simulink model "InterpolationIkinePD2019"  (R2019b)
settings: Solver=FixedStepDiscrete  StartTime=0.0  StopTime=inf  FixedStep=1/100  RelTol=1e-3
values from neighbouring files (symbols this model uses):
  Kd = 0.1    [LetterN.mat]    (also in initNew.m; panda.m)
  Kp = 10    [LetterN.mat]    (also in initNew.m; panda.m)
libraries: xpcutilitieslib x2, xpcrtudplib x2, robotcorelib x1, robotmaniplib x1, simulink x1
settings Model: EnablePacing=on  Creator=Aljaz  LastModifiedBy=jelac
settings DebuggingCC: ArithmeticOperatorsInVariantConditions=warning
settings SFSimCC: CustomCodeUndefinedFunction=UseInterfaceOnly
settings RTWCC: Toolchain=Microsoft Visual C++ 2019 v16.0 | nmake (64-bit Windows)

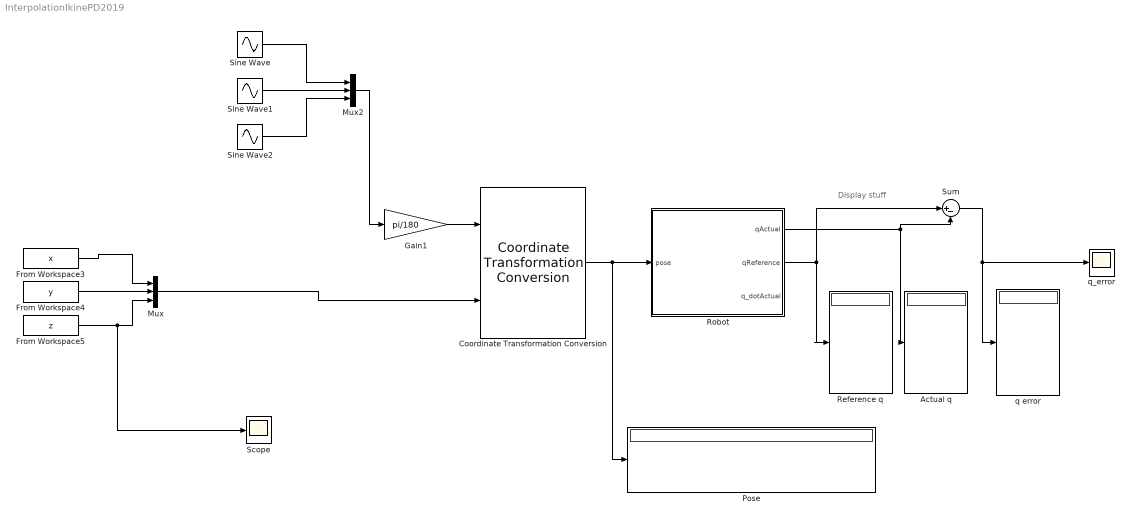
== system InterpolationIkinePD2019 ==
  note: Display stuff
  Actual q : Display
  Coordinate Transformation Conversion : robotcorelib/Coordinate Transformation Conversion  InputRepresentation=Euler Angles  InputEulerSequence=ZYX  ShowTrVecInputPort=on  OutputRepresentation=Homogeneous Transformation  OutputEulerSequence=ZYX  ShowTrVecOutputPort=on  SimulateUsing=Interpreted execution
      settings: SourceProductBaseCode=NV,RO,RR
  From Workspace3 : FromWorkspace  VariableName=x  SampleTime=0.01
  From Workspace4 : FromWorkspace  VariableName=y  SampleTime=0.01
  From Workspace5 : FromWorkspace  VariableName=z  SampleTime=0.01
  Gain1 : Gain  Gain=pi/180
  Mux : Mux  Inputs=3
  Mux2 : Mux  Inputs=3
  Pose : Display
  Reference q : Display
  Robot : Subsystem
  Scope : Scope
  Sine Wave : Sin  Amplitude=15  SampleTime=0
  Sine Wave1 : Sin  Amplitude=10  SampleTime=0
  Sine Wave2 : Sin  Amplitude=5  Bias=180  SampleTime=0
  Sum : Sum  Inputs=|+-
  q error : Display
  q_error : Scope
  wires:
  Robot/1(qActual) -> Sum/2, Actual q/1
  Robot/2(qReference) -> Sum/1, Reference q/1
  Coordinate Transformation Conversion/1 -> Pose/1, Robot/1(pose)
  Mux/1 -> Coordinate Transformation Conversion/2
  Sum/1 -> q_error/1, q error/1
  From Workspace3/1 -> Mux/1
  From Workspace4/1 -> Mux/2
  From Workspace5/1 -> Scope/1, Mux/3
  Sine Wave2/1 -> Mux2/3
  Sine Wave/1 -> Mux2/1
  Sine Wave1/1 -> Mux2/2
  Mux2/1 -> Gain1/1
  Gain1/1 -> Coordinate Transformation Conversion/1

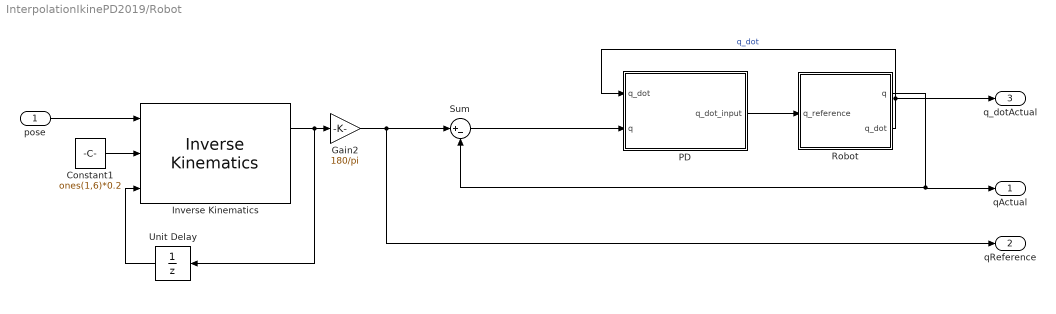
== system InterpolationIkinePD2019/Robot ==
  pose : Inport
  Constant1 : Constant  Value=ones(1,6)*0.2
  Gain2 : Gain  Gain=180/pi
  Inverse Kinematics : robotmaniplib/Inverse Kinematics  RigidBodyTree=robot  EndEffector=panda_hand  ShowInfo=on  SolverName=BFGS Gradient Projection  EnforceJointLimits=on  MaxIterations=250  MaxTime=inf  GradientTolerance=1e-7  SolutionTolerance=1e-6  StepTolerance=1e-6  ErrorChangeTolerance=1e-6  UseErrorDamping=on  DampingBias=0.0025  SimulateUsing=Code generation
  PD : Subsystem
  Robot : Subsystem
  Sum : Sum  Inputs=|+-
  Unit Delay : UnitDelay  InitialCondition=[0 0 0 -1.5708 0 1.5708 0]'  SampleTime=-1  HasFrameUpgradeWarning=on
  qActual : Outport
  qReference : Outport  Port=2
  q_dotActual : Outport  Port=3
  wires:
  Robot/1(q) -> qActual/1, Sum/2
  Inverse Kinematics/1 -> Unit Delay/1, Gain2/1
  pose/1 -> Inverse Kinematics/1
  Constant1/1 -> Inverse Kinematics/2
  Gain2/1 -> qReference/1, Sum/1
  Unit Delay/1 -> Inverse Kinematics/3
  Robot/2(q_dot) -> q_dotActual/1, PD/1(q_dot)  "q_dot"
  Sum/1 -> PD/2(q)
  PD/1(q_dot_input) -> Robot/1(q_reference)

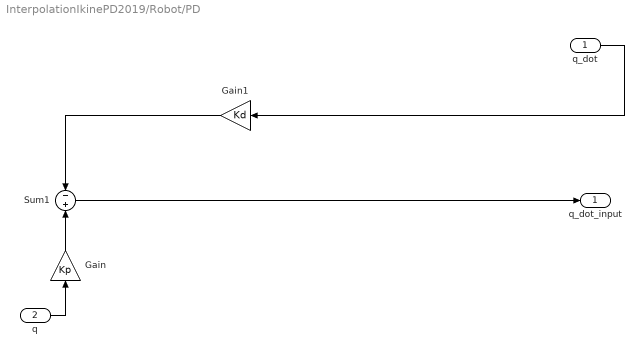
== system InterpolationIkinePD2019/Robot/PD ==
  q_dot : Inport
  q : Inport  Port=2
  Gain : Gain  Gain=Kp
  Gain1 : Gain  Gain=Kd
  Sum1 : Sum  Inputs=-|+
  q_dot_input : Outport
  wires:
  q/1 -> Gain/1
  q_dot/1 -> Gain1/1
  Gain1/1 -> Sum1/1
  Gain/1 -> Sum1/2
  Sum1/1 -> q_dot_input/1

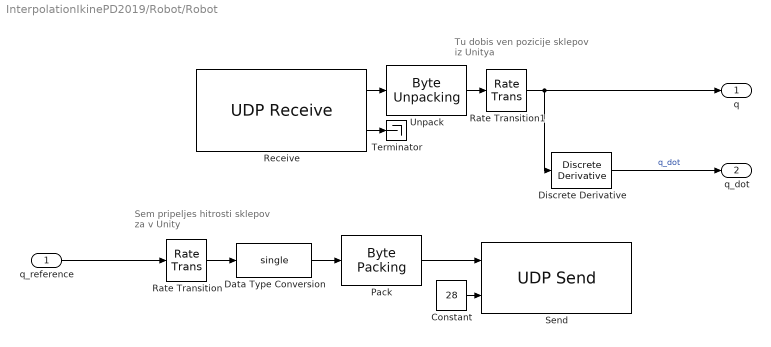
== system InterpolationIkinePD2019/Robot/Robot ==
  note: Sem pripeljes hitrosti sklepov za v Unity
  note: Tu dobis ven pozicije sklepov iz Unitya
  q_reference : Inport
  Constant : Constant  Value=28
  Data Type Conversion : DataTypeConversion  OutDataTypeStr=single
  Discrete Derivative : simulink/Discrete/Discrete Derivative  gainval=1  ICPrevScaledInput=0.0  OutMin=[]  OutMax=[]  OutDataType=fixdt(1, 16)  OutScaling=2^-10  DoSatur=off
  Pack : xpcutilitieslib/Byte Packing   MaskPackedDataType=uint8  MaskUnpackedDataTypes={'single'}  MaskAlignment=1
  Rate Transition : RateTransition  InitialCondition=[0 0 0 0 0 0 0]
  Rate Transition1 : RateTransition
  Receive : xpcrtudplib/UDP Receive  ipAddressVal=Use host-target connection  localPort=25106  rcvWidth=7*4  rcvFmAny=off  fmAddress=127.0.0.1  rcvMulticast=off  multicastAddress={}  maxUDPQueue=8  sampleTime=0.01
  Send : xpcrtudplib/UDP Send  ipAddressVal=Use host-target connection  localPort=-1  toAddress=127.0.0.1  toPort=25008  sampleTime=0.01
      settings: SourceProductBaseCode=XP
  Terminator : Terminator
  Unpack : xpcutilitieslib/Byte Unpacking   MaskUnpackedDataTypes={'single'}  MaskUnpackedDataSizes={[7]}  MaskAlignment=1
      settings: SourceProductBaseCode=XP
  q : Outport
  q_dot : Outport  Port=2
  wires:
  Constant/1 -> Send/2
  Pack/1 -> Send/1
  Receive/1 -> Unpack/1
  Rate Transition/1 -> Data Type Conversion/1
  Unpack/1 -> Rate Transition1/1
  Receive/2 -> Terminator/1
  Data Type Conversion/1 -> Pack/1
  Discrete Derivative/1 -> q_dot/1  "q_dot"
  q_reference/1 -> Rate Transition/1
  Rate Transition1/1 -> q/1, Discrete Derivative/1
